simulink model "examination"  (R2015b)
settings: Solver=VariableStepAuto  StartTime=0.0  StopTime=inf  RelTol=1e-3
libraries: robotlib x8
settings Model: Creator=weberhsu  LastModifiedBy=weberhsu

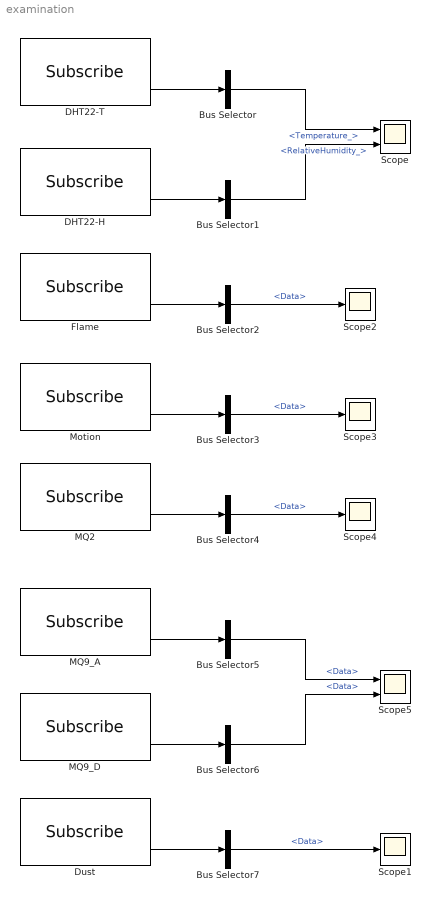
== system examination ==
  Bus Selector : BusSelector  OutputSignals=Temperature_
  Bus Selector1 : BusSelector  OutputSignals=RelativeHumidity_
  Bus Selector{2..7} (6 alike) : BusSelector  OutputSignals=Data
  DHT22-H : robotlib/Subscribe  SourceLibraryInfo=This block requires Robotics System Toolbox  topicSource=Select from ROS network  topic=/CurHumidity  messageType=sensor_msgs/RelativeHumidity  sampleTime=-1  messageQueueLength=1
  DHT22-T : robotlib/Subscribe  SourceLibraryInfo=This block requires Robotics System Toolbox  topicSource=Select from ROS network  topic=/CurTemperature  messageType=sensor_msgs/Temperature  sampleTime=-1  messageQueueLength=1
  Dust : robotlib/Subscribe  SourceLibraryInfo=This block requires Robotics System Toolbox  topicSource=Select from ROS network  topic=/DustDetection  messageType=std_msgs/Float32  sampleTime=-1  messageQueueLength=1
  Flame : robotlib/Subscribe  SourceLibraryInfo=This block requires Robotics System Toolbox  topicSource=Select from ROS network  topic=/FlameDetectionDistance  messageType=std_msgs/Float32  sampleTime=-1  messageQueueLength=1
  MQ2 : robotlib/Subscribe  SourceLibraryInfo=This block requires Robotics System Toolbox  topicSource=Select from ROS network  topic=/SmokeDetectionMQ2  messageType=std_msgs/Float32  sampleTime=-1  messageQueueLength=1
  MQ9_A : robotlib/Subscribe  SourceLibraryInfo=This block requires Robotics System Toolbox  topicSource=Select from ROS network  topic=/SmokeDetectionMQ9_A  messageType=std_msgs/Float32  sampleTime=-1  messageQueueLength=1
  MQ9_D : robotlib/Subscribe  SourceLibraryInfo=This block requires Robotics System Toolbox  topicSource=Select from ROS network  topic=/SmokeDetectionMQ9_D  messageType=std_msgs/Bool  sampleTime=-1  messageQueueLength=1
  Motion : robotlib/Subscribe  SourceLibraryInfo=This block requires Robotics System Toolbox  topicSource=Select from ROS network  topic=/MotionDetection  messageType=std_msgs/Bool  sampleTime=-1  messageQueueLength=1
  Scope : Scope  NumInputPorts=2
  Scope{1..4} (4 alike) : Scope
  Scope5 : Scope  NumInputPorts=2
  wires:
  DHT22-T/2 -> Bus Selector/1
  Bus Selector/1 -> Scope/1  "<Temperature_>"
  DHT22-H/2 -> Bus Selector1/1
  Bus Selector1/1 -> Scope/2  "<RelativeHumidity_>"
  Flame/2 -> Bus Selector2/1
  Bus Selector2/1 -> Scope2/1  "<Data>"
  Motion/2 -> Bus Selector3/1
  Bus Selector3/1 -> Scope3/1  "<Data>"
  MQ2/2 -> Bus Selector4/1
  Bus Selector4/1 -> Scope4/1  "<Data>"
  MQ9_A/2 -> Bus Selector5/1
  Bus Selector5/1 -> Scope5/1  "<Data>"
  MQ9_D/2 -> Bus Selector6/1
  Bus Selector6/1 -> Scope5/2  "<Data>"
  Dust/2 -> Bus Selector7/1
  Bus Selector7/1 -> Scope1/1  "<Data>"
